simulink model "Altitude_AirSpeed_hold_Sim"  (R2016b)
settings: Solver=VariableStepAuto  StartTime=0.0  StopTime=100  RelTol=1e-3
values from neighbouring files (symbols this model uses):
  A = [-0.0447 -0.0076 0.0293 0 0 0 5.6993 -1.4866 -12.1418 0 -50 0 ... (36 elements, 6x6)]    [B.mat]    (also in B_observer.mat; B_wind.mat; K.mat; K_observer.mat)
  A_observer = [-10.2335641808 0.0739061145334 -0.265410048349 -0.17408532662 -2.92649849477 -64661.8021967 5.6993 -1.4866 -12.1418 0 -50 0 ... (36 elements, 6x6)]    [A_observer.mat]    (also in B_observer.mat; matlab.mat)
  B_observer = [0 -0.3067 -40.6088 0 0 0 1.7371 -0.0025 -0.2448 0 0 706.5875 ... (24 elements, 6x4)]    [B_observer.mat]    (also in matlab.mat)
  B_wind = [0 -0.3067 -40.6088 0 0 0 1.7371 -0.0025 -0.2448 0 0 706.5875 ... (24 elements, 6x4)]    [B_wind.mat]    (also in matlab.mat)
  C = [1 0 0 0 0 0 0 1 0 0 0 0 ... (36 elements, 6x6)]    [B.mat]    (also in B_observer.mat = [1  0  0  0  0  0; 0  0  0  0  1  0]; B_wind.mat = [1  0  0  0  0  0; 0  0  0  0  1  0]; K.mat = [1  0  0  0  0  0; 0  0  0  0  1  0]; K_observer.mat = [1  0  0  0  0  0; 0  0  0  0  1  0])
  K = [0.0696040842818  1.49094912051  -0.0975947639883  -2.34467127052  -0.0472919275262  4.54349713499e-06; 0.155951603894  -0.447600306196  0.00298574492524  0.443772615641  0.0315082037392  9.49570961121e-05]    [B_observer.mat]    (also in B_wind.mat = [0.568603067096  6.84894626738  -0.267785637236  -9.62832121; K.mat = [0.568603067096  6.84894626738  -0.267785637236  -9.62832121; K_observer.mat; N_uy.mat = [0.568603067096  6.84894626738  -0.267785637236  -9.62832121)
  Kf = [0.0551192592558  -0.0208594511839; 0.0278126015785  0.00459327160465]    [B_observer.mat]    (also in B_wind.mat = [0.527353058781  -0.212411562685; 0.283215416913  0.04394608; K.mat = [0.527353058781  -0.212411562685; 0.283215416913  0.04394608; K_observer.mat; N_uy.mat = [0.527353058781  -0.212411562685; 0.283215416913  0.04394608)
  N_uy_bar = [0.0023441981438  0; 0.00913644457561  0]    [B_observer.mat]    (also in B_wind.mat; K.mat; K_observer.mat; N_uy.mat)
libraries: simulink x2
settings Model: Creator=Santi  LastModifiedBy=Santi

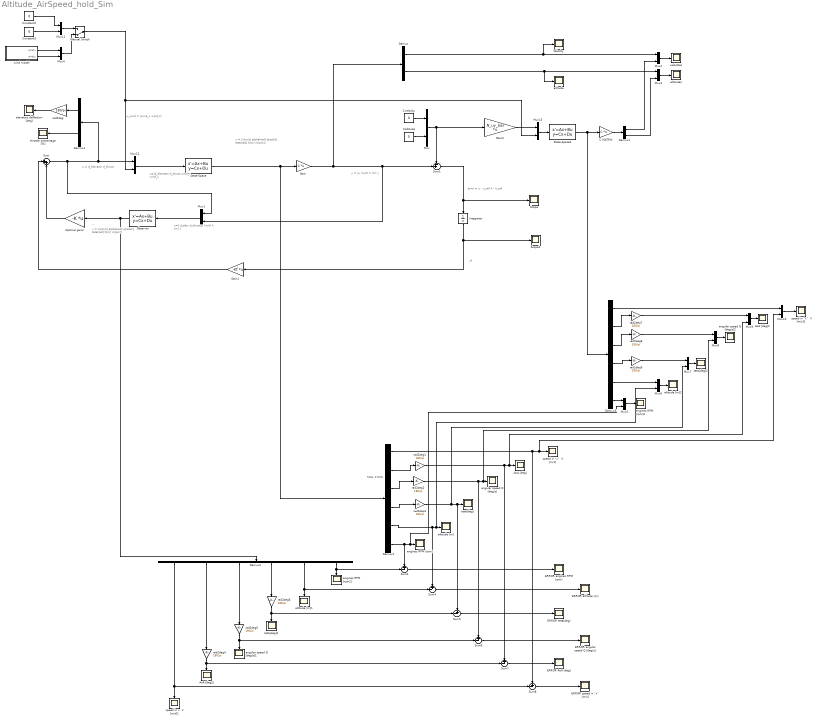
== system Altitude_AirSpeed_hold_Sim ==
  note: yf
  note: u=[d_elevator
      | d_thrust
      | wind_x
      | wind_z
  note: u=[ d_elev
      |       d_thrust
      |       u (m/s)
      |       h (m) ]
  note: u_wind = [wind_x
      |                 wind_z]
  note: error = u - u_ref
      | h - h_ref
  note: ^
  note: u = d_elevator
      | d_thrust
  note: y = [u (m/s)
      | h (m) ]
  note: x = [u[m/s]
      | alpha[rad]
      | q[rad/s]
      | teta[rad]
      | h[m]
      | n[rpm]]
  note: REAL STATE
  note: x = [u[m/s]
      | alpha[rad]
      | q[rad/s]
      | teta[rad]
      | h[m]
      | n[rpm]]
  AoA [deg] : Scope
  AoA [deg]1 : Scope
  AoA [deg]2 : Scope
  C MATRIX : Gain  Gain=C  Multiplication=Matrix(K*u)
  Caltitude : Constant  Value=5
  Constant2 : Constant  Value=0
  Constant3 : Constant  Value=0
  Cvelocity : Constant  Value=0
  Demux : Demux  Outputs=2
  Demux1 : Demux  Outputs=2
  Demux2 : Demux  Outputs=6
  Demux3 : Demux  Outputs=6
  Demux4 : Demux  Outputs=2
  Demux5 : Demux  Outputs=6
  ERROR AoA [deg] : Scope
  ERROR altitude [m] : Scope
  ERROR engines RPM [rpm] : Scope
  ERROR teta[deg] : Scope
  ERROR angular speed Q [deg/s] : Scope
  "ERROR speed in \"x\"  [m/s]" : Scope
  Gain : Gain  Gain=C  Multiplication=Matrix(K*u)
  Gain1 : Gain  Gain=-Kf  Multiplication=Matrix(K*u)
  Gain3 : Gain  Gain=N_uy_bar  Multiplication=Matrix(K*u)
  Integrator : Integrator
  Manual Switch : ManualSwitch  CurrentSetting=0
  Mux{,1..13} (14 alike) : Mux  Inputs=2
  Observer : StateSpace  A=A_observer  B=B_observer  C=eye(6)  D=zeros(6,4)  X0=[0 0 0 0 0 0]
  Optimal ganin : Gain  Gain=-K  Multiplication=Matrix(K*u)
  Scope : Scope
  Scope2 : Scope
  State-Space : StateSpace  A=A  B=B_wind  C=eye(6)  D=zeros(6,4)  X0=[1 0 0 0 0 0]
  State-Space2 : StateSpace  A=A  B=B_wind  C=eye(6)  D=zeros(6,4)  X0=[1 0 0 0 0 0]
  Sum : Sum  Inputs=|++
  Sum1 : Sum  Inputs=-+|
  Sum{3..8} (6 alike) : Sum  Inputs=+-|
  Velocity : Scope
  altitude : Scope
  altitude [m] : Scope
  altitude [m]1 : Scope
  altitude [m]2 : Scope
  altitudes : Scope
  angular speed Q [deg/s] : Scope
  angular speed Q [deg/s]1 : Scope
  angular speed Q [deg/s]2 : Scope
  elevators deflection [deg] : Scope
  engines RPM [rpm] : Scope
  engines RPM [rpm]1 : Scope
  engines RPM [rpm]2 : Scope
  rad2deg{,1..9} (10 alike) : Gain  Gain=180/pi
  speed in x  V [m/s]1 : Scope
  "speed in \"x\"  V [m/s]" : Scope
  "speed in \"x\"  V [m/s]1" : Scope
  teta[deg] : Scope
  teta[deg]1 : Scope
  teta[deg]2 : Scope
  throttle precentage [%] : Scope
  velocities : Scope
  wind model : Subsystem  TreatAsAtomicUnit=on
  wires:
  Gain1/1 -> Sum/1
  Optimal ganin/1 -> Sum/2
  Sum1/1 -> Scope/1, Integrator/1
  Gain/1 -> Sum1/2, Mux1/2, Demux/1
  Integrator/1 -> Scope2/1, Gain1/1
  Caltitude/1 -> Mux/2
  Cvelocity/1 -> Mux/1
  Mux/1 -> Gain3/1, Sum1/1
  Demux/2 -> altitude/1, Mux3/1
  Demux/1 -> Velocity/1, Mux2/1
  Mux1/1 -> Observer/1
  C MATRIX/1 -> Demux1/1
  Demux1/1 -> Mux2/2
  Demux1/2 -> Mux3/2
  Mux3/1 -> altitudes/1
  Mux2/1 -> velocities/1
  State-Space/1 -> Gain/1, Demux3/1
  Demux3/6 -> Mux5/2, engines RPM [rpm]/1, Sum3/1
  Demux3/5 -> Mux6/2, altitude [m]/1, Sum4/1
  rad2deg2/1 -> Mux8/2, angular speed Q [deg/s]/1, Sum6/1
  rad2deg1/1 -> Mux9/2, AoA [deg]/1, Sum7/1
  Demux3/1 -> Mux10/2, "speed in \"x\"  V [m/s]"/1, Sum8/1
  Demux3/2 -> rad2deg1/1
  Demux3/3 -> rad2deg2/1
  Demux3/4 -> rad2deg3/1
  Observer/1 -> Optimal ganin/1, Demux2/1
  Demux2/6 -> Sum3/2, engines RPM [rpm]1/1
  Demux2/5 -> Sum4/2, altitude [m]1/1
  rad2deg6/1 -> Sum5/2, teta[deg]1/1
  rad2deg5/1 -> Sum6/2, angular speed Q [deg/s]1/1
  rad2deg4/1 -> AoA [deg]1/1, Sum7/2
  Demux2/1 -> Sum8/2, speed in x  V [m/s]1/1
  Demux2/2 -> rad2deg4/1
  Demux2/3 -> rad2deg5/1
  Demux2/4 -> rad2deg6/1
  Sum3/1 -> ERROR engines RPM [rpm]/1
  Sum4/1 -> ERROR altitude [m]/1
  Sum5/1 -> ERROR teta[deg]/1
  Sum6/1 -> ERROR angular speed Q [deg/s]/1
  Sum7/1 -> ERROR AoA [deg]/1
  Sum8/1 -> "ERROR speed in \"x\"  [m/s]"/1
  rad2deg3/1 -> Mux7/2, teta[deg]/1, Sum5/1
  State-Space2/1 -> Demux5/1, C MATRIX/1
  Demux5/6 -> Mux5/1
  Demux5/5 -> Mux6/1
  rad2deg8/1 -> Mux8/1
  rad2deg7/1 -> Mux9/1
  Demux5/1 -> Mux10/1
  Demux5/2 -> rad2deg7/1
  Demux5/3 -> rad2deg8/1
  Demux5/4 -> rad2deg9/1
  rad2deg9/1 -> Mux7/1
  Mux10/1 -> "speed in \"x\"  V [m/s]1"/1
  Mux9/1 -> AoA [deg]2/1
  Mux8/1 -> angular speed Q [deg/s]2/1
  Mux7/1 -> teta[deg]2/1
  Mux6/1 -> altitude [m]2/1
  Mux5/1 -> engines RPM [rpm]2/1
  rad2deg/1 -> elevators deflection [deg]/1
  Demux4/1 -> rad2deg/1
  Demux4/2 -> throttle precentage [%]/1
  Sum/1 -> Mux1/1, Demux4/1, Mux12/1
  wind model/1(wind x) -> Mux4/1
  wind model/2(wind z) -> Mux4/2
  Constant3/1 -> Mux11/2
  Constant2/1 -> Mux11/1
  Mux11/1 -> Manual Switch/1
  Mux4/1 -> Manual Switch/2
  Mux12/1 -> State-Space/1
  Manual Switch/1 -> Mux12/2, Mux13/2
  Mux13/1 -> State-Space2/1
  Gain3/1 -> Mux13/1

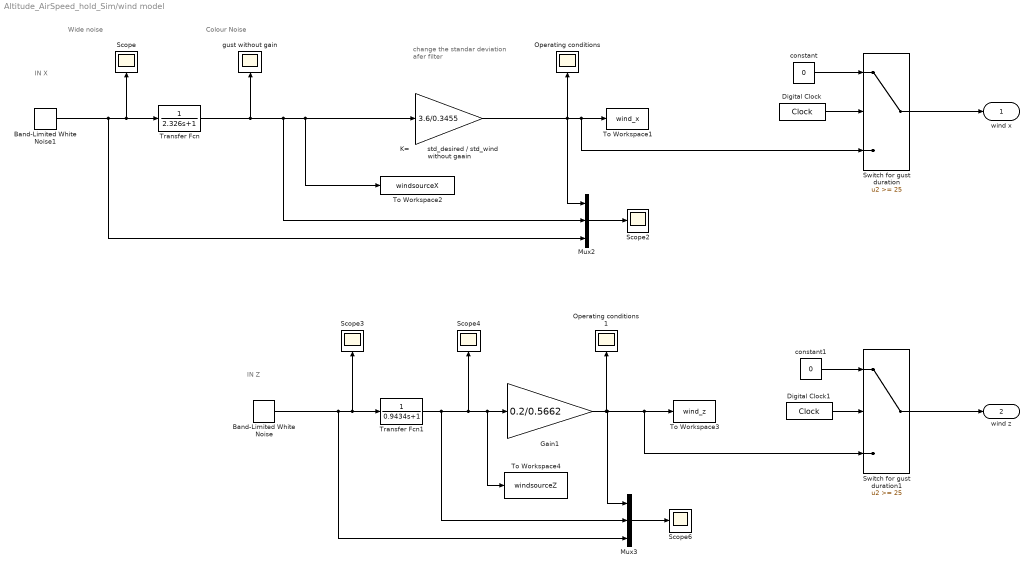
== system Altitude_AirSpeed_hold_Sim/wind model ==
  note: change the standar deviation afer filter
  note: Colour Noise
  note: Wide noise
  note: IN Z
  note: IN X
  Band-Limited White Noise : simulink/Sources/Band-Limited White Noise  Cov=[0.7]  Ts=0.1  seed=[23341]
  Band-Limited White Noise1 : simulink/Sources/Band-Limited White Noise  Cov=[0.7]  Ts=0.1  seed=[23341]
  Digital Clock : DigitalClock
  Digital Clock1 : DigitalClock
  Gain1 : Gain  Gain=0.2/0.5662
  K=         std_desired / std_wind without gaain : Gain  Gain=3.6/0.3455
  Mux2 : Mux  Inputs=3
  Mux3 : Mux  Inputs=3
  "Operating conditions " : Scope
  Operating conditions 1 : Scope
  Scope{,2..4,6} (5 alike) : Scope
  Switch for gust duration : Switch  Threshold=25
  Switch for gust duration1 : Switch  Threshold=25
  To Workspace1 : ToWorkspace  VariableName=wind_x  SampleTime=-1
  To Workspace2 : ToWorkspace  VariableName=windsourceX  SampleTime=-1
  To Workspace3 : ToWorkspace  VariableName=wind_z  SampleTime=-1
  To Workspace4 : ToWorkspace  VariableName=windsourceZ  SampleTime=-1
  Transfer Fcn : TransferFcn  Denominator=[2.326 1]
  Transfer Fcn1 : TransferFcn  Denominator=[0.9434 1]
  constant : Constant  Value=0
  constant1 : Constant  Value=0
  gust without gain : Scope
  wind x : Outport
  wind z : Outport  Port=2
  wires:
  Transfer Fcn/1 -> K=         std_desired / std_wind without gaain/1, To Workspace2/1, Mux2/2, gust without gain/1
  K=         std_desired / std_wind without gaain/1 -> "Operating conditions "/1, Mux2/1, Switch for gust duration/3, To Workspace1/1
  Switch for gust duration/1 -> wind x/1
  Digital Clock/1 -> Switch for gust duration/2
  constant/1 -> Switch for gust duration/1
  Switch for gust duration1/1 -> wind z/1
  Digital Clock1/1 -> Switch for gust duration1/2
  constant1/1 -> Switch for gust duration1/1
  Band-Limited White Noise1/1 -> Mux2/3, Transfer Fcn/1, Scope/1
  Mux2/1 -> Scope2/1
  Transfer Fcn1/1 -> Mux3/2, Gain1/1, To Workspace4/1, Scope4/1
  Gain1/1 -> Operating conditions 1/1, Mux3/1, To Workspace3/1, Switch for gust duration1/3
  Band-Limited White Noise/1 -> Mux3/3, Scope3/1, Transfer Fcn1/1
  Mux3/1 -> Scope6/1
